simulink model "test03_mod05"  (Simulink 7.4)
settings: Solver=FixedStepDiscrete  SolverMode=SingleTasking  StartTime=0.0  StopTime=inf  FixedStep=0.01  RelTol=1e-3  SampleTimeConstraint=Specified
undefined symbols (not defined in the file or in its folder): serial
libraries: instrumentlib x2, simulink x1
settings Model: Creator=Administrateur  LastModifiedBy=djulzz
settings MATStruct: SampleTime=0.1  Offset=0  Priority=[10.0]

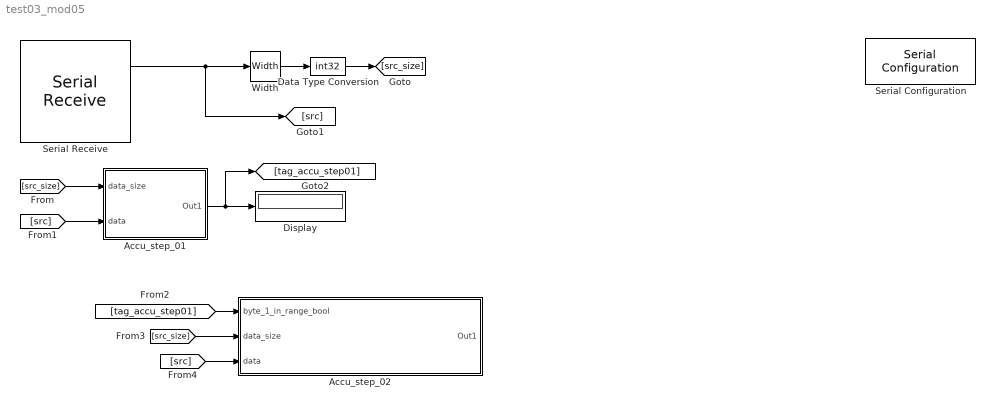
== system test03_mod05 ==
  Accu_step_01 : Subsystem
  Accu_step_02 : Subsystem
  Data Type Conversion : DataTypeConversion  OutDataTypeMode=int32  OutDataType=fixdt(1, 16)  OutScaling=2^0  OutDataTypeStr=int32
  Display : Display
  Serial Configuration : instrumentlib/Serial Configuration  Priority=-200000  DialogController=instrumentcreatedialog  DialogControllerArgs=DataTag0  ComPortMenu=<Please select a port...>  ComPort=COM4  ObjConstructor=serial('COM4');  BaudRate=38400  DataBits=8  Parity=none  StopBits=1  FlowControl=none  Timeout=10  ByteOrder=LittleEndian
  Serial Receive : instrumentlib/Serial Receive  DialogController=instrumentcreatedialog  DialogControllerArgs=DataTag1  ComPortMenu=<Please select a port...>  ComPort=COM4  ObjConstructor=serial('COM4');  Terminator=<none>  DataSize="[40   1]"  DataType=uint8  EnableBlockingMode=off  ActionDataUnavailable=Output last received value  CustomValue=0  SampleTime=-1
  Width : Width
  wires:
  Width/1 -> Data Type Conversion/1
  Data Type Conversion/1 -> [src_size]
  Serial Receive/1 -> Width/1, [src]
  [src_size] -> Accu_step_01/1(data_size)
  [src] -> Accu_step_01/2(data)
  Accu_step_01/1(Out1) -> Display/1, [tag_accu_step01]
  [tag_accu_step01] -> Accu_step_02/1(byte_1_in_range_bool)
  [src_size] -> Accu_step_02/2(data_size)
  [src] -> Accu_step_02/3(data)

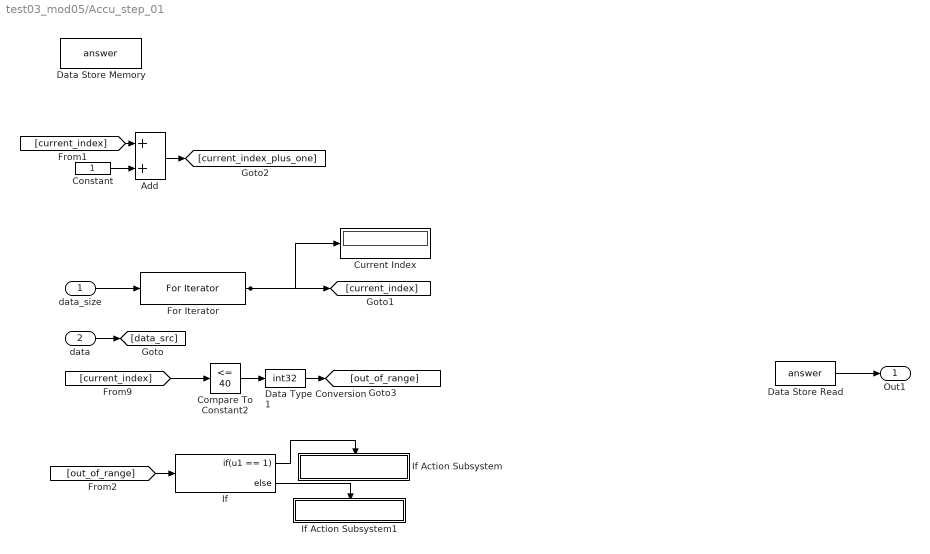
== system test03_mod05/Accu_step_01 ==
  data_size : Inport  DataType=int32  OutDataType=fixdt(1, 16)  OutScaling=2^0  OutDataTypeStr=int32
  data : Inport  Port=2  DataType=uint8  OutDataType=fixdt(1, 16)  OutScaling=2^0  OutDataTypeStr=uint8
  Add : Sum  AccumDataTypeStr=int32  OutDataTypeMode=int32  OutDataType=fixdt(1, 16)  OutScaling=2^-10  OutDataTypeStr=int32
  Compare To Constant2 : simulink/Logic and Bit Operations/Compare To Constant  SystemSampleTime=-1  relop=<=  const=40  LogicOutDataTypeMode=boolean  ZeroCross=off
  Constant : Constant  OutDataTypeMode=int32  OutDataType=fixdt(1, 16)  OutScaling=2^0  OutDataTypeStr=int32  SampleTime=-1
  Current Index : Display
  Data Store Memory : DataStoreMemory  DataStoreName=answer  DataType=int32  OutDataType=fixdt(1, 16)  OutScaling=2^0  OutDataTypeStr=int32
  Data Store Read : DataStoreRead  DataStoreName=answer  SampleTime=-1
  Data Type Conversion1 : DataTypeConversion  OutDataTypeMode=int32  OutDataType=fixdt(1, 16)  OutScaling=2^0  OutDataTypeStr=int32
  For Iterator : ForIterator  IterationSource=external
  If : If  IfExpression=u1 == 1
  If Action Subsystem : Subsystem  TreatAsAtomicUnit=on
  If Action Subsystem1 : Subsystem  TreatAsAtomicUnit=on
  Out1 : Outport  DataType=int32  OutDataType=fixdt(1, 16)  OutScaling=2^0  OutDataTypeStr=int32
  wires:
  data_size/1 -> For Iterator/1
  data/1 -> [data_src]
  For Iterator/1 -> [current_index], Current Index/1
  Constant/1 -> Add/2
  [current_index] -> Add/1
  Add/1 -> [current_index_plus_one]
  Compare To Constant2/1 -> Data Type Conversion1/1
  Data Type Conversion1/1 -> [out_of_range]
  [current_index] -> Compare To Constant2/1
  [out_of_range] -> If/1
  If/2 -> If Action Subsystem1/Action
  If/1 -> If Action Subsystem/Action
  Data Store Read/1 -> Out1/1

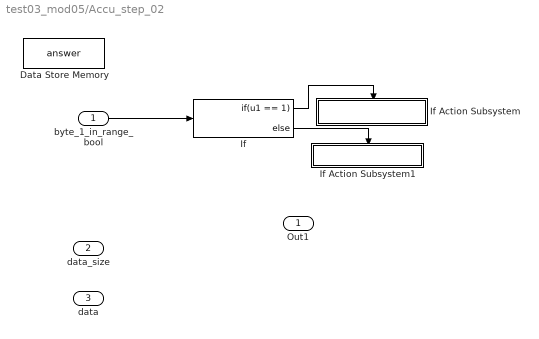
== system test03_mod05/Accu_step_02 ==
  byte_1_in_range_bool : Inport  DataType=int32  OutDataType=fixdt(1, 16)  OutScaling=2^0  OutDataTypeStr=int32
  data_size : Inport  Port=2  DataType=int32  OutDataType=fixdt(1, 16)  OutScaling=2^0  OutDataTypeStr=int32
  data : Inport  Port=3  DataType=uint8  OutDataType=fixdt(1, 16)  OutScaling=2^0  OutDataTypeStr=uint8
  Data Store Memory : DataStoreMemory  DataStoreName=answer  DataType=int32  OutDataType=fixdt(1, 16)  OutScaling=2^0  OutDataTypeStr=int32
  If : If  IfExpression=u1 == 1
  If Action Subsystem : Subsystem  TreatAsAtomicUnit=on
  If Action Subsystem1 : Subsystem  TreatAsAtomicUnit=on
  Out1 : Outport  OutDataType=fixdt(1, 16)  OutScaling=2^0
  wires:
  byte_1_in_range_bool/1 -> If/1
  If/2 -> If Action Subsystem1/Action
  If/1 -> If Action Subsystem/Action

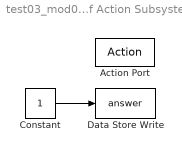
== system test03_mod05/Accu_step_01/If Action Subsystem ==
  Action Port : ActionPort  PropagateVarSize=During execution  ActionType=then
  Constant : Constant  OutDataTypeMode=int32  OutDataType=fixdt(1, 16)  OutScaling=2^0  OutDataTypeStr=int32  SampleTime=-1
  Data Store Write : DataStoreWrite  DataStoreName=answer  SampleTime=-1
  wires:
  Constant/1 -> Data Store Write/1

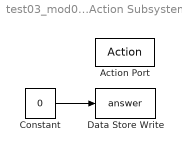
== system test03_mod05/Accu_step_01/If Action Subsystem1 ==
  Action Port : ActionPort  PropagateVarSize=During execution  ActionType=else
  Constant : Constant  Value=0  OutDataTypeMode=int32  OutDataType=fixdt(1, 16)  OutScaling=2^0  OutDataTypeStr=int32  SampleTime=-1
  Data Store Write : DataStoreWrite  DataStoreName=answer  SampleTime=-1
  wires:
  Constant/1 -> Data Store Write/1

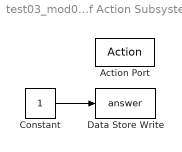
== system test03_mod05/Accu_step_02/If Action Subsystem ==
  Action Port : ActionPort  PropagateVarSize=During execution  ActionType=then
  Constant : Constant  OutDataTypeMode=int32  OutDataType=fixdt(1, 16)  OutScaling=2^0  OutDataTypeStr=int32  SampleTime=-1
  Data Store Write : DataStoreWrite  DataStoreName=answer  SampleTime=-1
  wires:
  Constant/1 -> Data Store Write/1

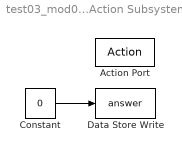
== system test03_mod05/Accu_step_02/If Action Subsystem1 ==
  Action Port : ActionPort  PropagateVarSize=During execution  ActionType=else
  Constant : Constant  Value=0  OutDataTypeMode=int32  OutDataType=fixdt(1, 16)  OutScaling=2^0  OutDataTypeStr=int32  SampleTime=-1
  Data Store Write : DataStoreWrite  DataStoreName=answer  SampleTime=-1
  wires:
  Constant/1 -> Data Store Write/1
